simulink model "CANTXcommunicationunit"  (R2024a)
settings: Solver=VariableStepAuto  StartTime=0.0  StopTime=10.0  RelTol=1e-3
undefined symbols (not defined in the file or in its folder): canChannel
libraries: canlib x3, canmsglib x2
settings Model: DataDictionary=BMS_System_dict1.sldd  Creator=hirah  LastModifiedBy=hirah

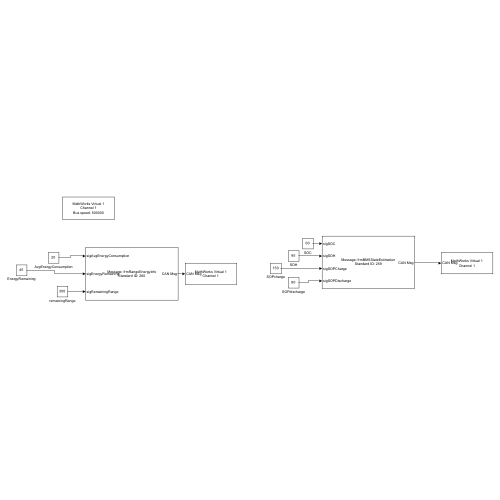
[thumbnail: Simulink's stored preview of the top-level diagram]
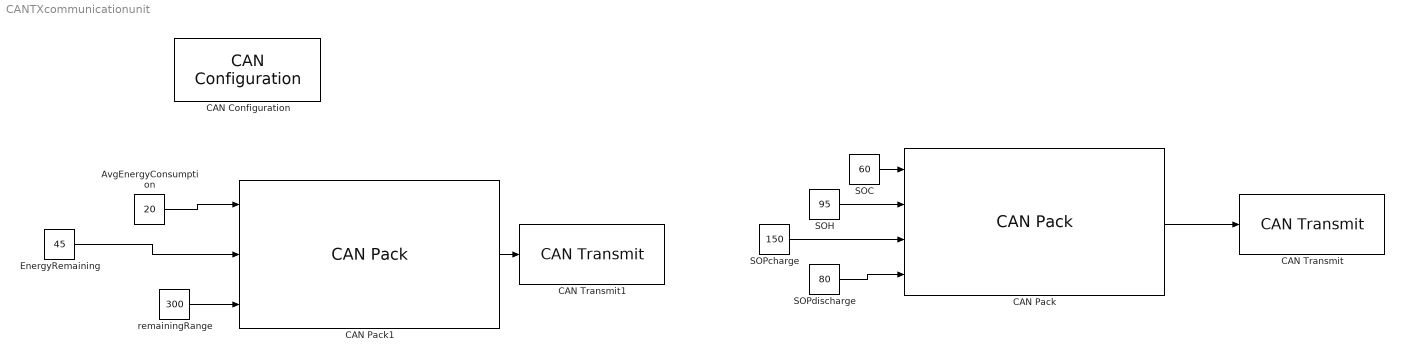
== system CANTXcommunicationunit ==
  AvgEnergyConsumption : Constant  Value=20  OutDataTypeStr=double
  CAN Configuration : canlib/CAN Configuration  BlockHandle=905.0004  Device=MathWorks Virtual 1 (Channel 1)  DeviceMenu=MathWorks Virtual 1 (Channel 1)  ObjConstructor=canChannel('MathWorks', 'Virtual 1', 1)  BusSpeed=500000  EnableBitParameters=off  AckMode=Normal
  CAN Pack : canmsglib/CAN Pack  CANdbFile=C:\Users\hirah\Downloads\BMS_CAN_Database (5).dbc  MsgList=frmBMSStateEstimation  MsgName=frmBMSStateEstimation  MsgIDType=Standard (11-bit identifier)  MsgIdentifier=259  MsgLength=6  Remote=off  ApplyMinMax=off  BusOutput=off  SignalInfo={ 'sigSOC', '0', '8', 'LE', 'unsigned', 'Standard', '0', '1', '0', '0', '100'; 'sigSOH', '8', '8', 'LE', 'unsigned', 'Standard', '0', '1', '0', '0', '100'; 'sigSOPCharge', '32', '16', 'LE', 'unsigned', 'Standard', '0', '1', '0', '0', '200'; 'sigSOPDischarge', '16', '16', 'LE', 'unsigned', 'Standard', '0', '1', '0', '0', '200' }
      settings: LibrarySourceBlock=canlib/CAN Pack  DataFormat=manually specified signals
  CAN Pack1 : canmsglib/CAN Pack  CANdbFile=C:\Users\hirah\Downloads\BMS_CAN_Database (5).dbc  MsgList=frmRangeEnergyInfo  MsgName=frmRangeEnergyInfo  MsgIDType=Standard (11-bit identifier)  MsgIdentifier=260  MsgLength=6  Remote=off  ApplyMinMax=off  BusOutput=off  SignalInfo={ 'sigAvgEnergyConsumption', '32', '16', 'LE', 'unsigned', 'Standard', '0', '0.01', '0', '0', '50'; 'sigEnergyRemaining', '16', '16', 'LE', 'unsigned', 'Standard', '0', '1', '0', '0', '200'; 'sigRemainingRange', '0', '16', 'LE', 'unsigned', 'Standard', '0', '1', '0', '0', '1000' }
      settings: LibrarySourceBlock=canlib/CAN Pack  DataFormat=manually specified signals
  CAN Transmit : canlib/CAN Transmit  BlockHandle=917.0001  Device=MathWorks Virtual 1 (Channel 1)  DeviceMenu=MathWorks Virtual 1 (Channel 1)  ObjConstructor=canChannel('MathWorks', 'Virtual 1', 1)  EnableEventTransmit=off  EnablePeriodicTransmit=off  MessagePeriod=1.000
  CAN Transmit1 : canlib/CAN Transmit  BlockHandle=919.0001  Device=MathWorks Virtual 1 (Channel 1)  DeviceMenu=MathWorks Virtual 1 (Channel 1)  ObjConstructor=canChannel('MathWorks', 'Virtual 1', 1)  EnableEventTransmit=off  EnablePeriodicTransmit=off  MessagePeriod=1.000
  EnergyRemaining : Constant  Value=45  OutDataTypeStr=uint16
  SOC : Constant  Value=60  OutDataTypeStr=uint8
  SOH : Constant  Value=95  OutDataTypeStr=uint8
  SOPcharge : Constant  Value=150  OutDataTypeStr=uint16
  SOPdischarge : Constant  Value=80  OutDataTypeStr=uint16
  remainingRange : Constant  Value=300  OutDataTypeStr=uint16
  wires:
  SOC/1 -> CAN Pack/1
  SOH/1 -> CAN Pack/2
  SOPcharge/1 -> CAN Pack/3
  SOPdischarge/1 -> CAN Pack/4
  CAN Pack/1 -> CAN Transmit/1
  AvgEnergyConsumption/1 -> CAN Pack1/1
  EnergyRemaining/1 -> CAN Pack1/2
  remainingRange/1 -> CAN Pack1/3
  CAN Pack1/1 -> CAN Transmit1/1
